simulink model "stopwatch_extended"  (R2020a)
settings: Solver=FixedStepAuto  StartTime=0.0  StopTime=1000.0  FixedStep=1e-3  RelTol=1e-3
settings Model: EnablePacing=on  Creator=Lukas Bilal  LastModifiedBy=Lukas Bilal

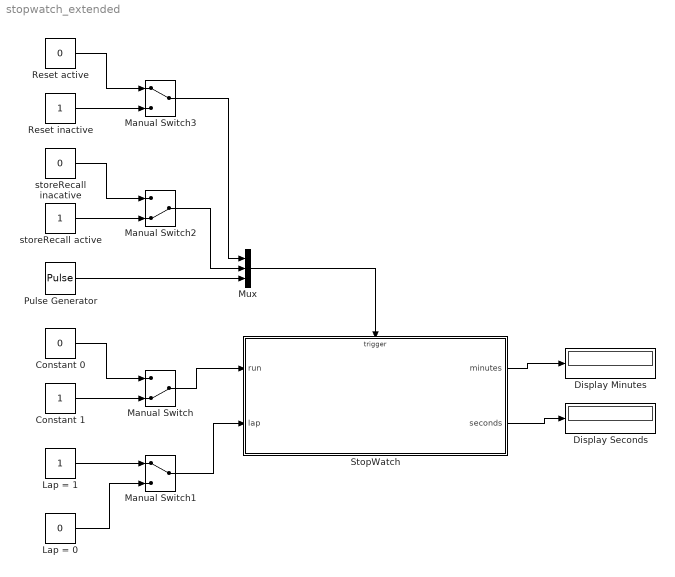
== system stopwatch_extended ==
  Constant 0 : Constant  Value=0  OutDataTypeStr=boolean
  Constant 1 : Constant  OutDataTypeStr=boolean
  Display Minutes : Display
  Display Seconds : Display
  Lap = 0 : Constant  Value=0  OutDataTypeStr=boolean
  Lap = 1 : Constant  OutDataTypeStr=boolean
  Manual Switch : ManualSwitch  CurrentSetting=0
  Manual Switch1 : ManualSwitch
  Manual Switch2 : ManualSwitch  CurrentSetting=0
  Manual Switch3 : ManualSwitch
  Mux : Mux  Inputs=3
  "Pulse Generator " : DiscretePulseGenerator  PulseType=Time based  Period=1  PulseWidth=5
  Reset active : Constant  Value=0  OutDataTypeStr=double
  Reset inactive : Constant  OutDataTypeStr=double
  StopWatch : Stateflow chart  TreatAsAtomicUnit=on
  storeRecall active : Constant  OutDataTypeStr=double
  storeRecall inacative : Constant  Value=0  OutDataTypeStr=double
  wires:
  "Pulse Generator "/1 -> Mux/3
  Constant 0/1 -> Manual Switch/1
  Constant 1/1 -> Manual Switch/2
  Manual Switch/1 -> StopWatch/1(run)
  StopWatch/1(minutes) -> Display Minutes/1
  StopWatch/2(seconds) -> Display Seconds/1
  Lap = 1/1 -> Manual Switch1/1
  Lap = 0/1 -> Manual Switch1/2
  Manual Switch1/1 -> StopWatch/2(lap)
  Mux/1 -> StopWatch/Trigger
  storeRecall inacative/1 -> Manual Switch2/1
  storeRecall active/1 -> Manual Switch2/2
  Manual Switch2/1 -> Mux/2
  Reset active/1 -> Manual Switch3/1
  Reset inactive/1 -> Manual Switch3/2
  Manual Switch3/1 -> Mux/1

== stateflow chart stopwatch_extended/StopWatch ==
  settings: executeAtInitialization=1
  state Stopped
    state Recall
    state Reset
    state Store
    (default) -> Recall
    Recall -> Reset [order 2] : Restart
    Store -> Recall [order 1] : storeRecall /
        | {
        |   minutes_intern = 0;
        |   seconds_intern = 0;
        |   seconds_stored = 0;
        |   minutes_stored = 0;
        | }
    Recall -> Store [order 1] : storeRecall /
        | {
        |   minutes_stored = minutes_intern;
        |   seconds_stored = seconds_intern;
        | }
    Reset -> Reset : {
        |   minutes_intern = 0;
        |   seconds_intern = 0;
        |   seconds_stored = 0;
        |   minutes_stored = 0;
        | }
    Store -> Reset [order 2] : Restart
  state Started
    state store_recall [parallel]
      settings: executionOrder=1
      (history)
      state recall
      state store
      (default) -> recall
      store -> recall : storeRecall /
          | {
          |   seconds_intern = seconds_stored;
          |   minutes_intern = minutes_stored;
          | }
      recall -> store : storeRecall /
          | {
          |   seconds_stored = seconds_intern;
          |   minutes_stored = minutes_intern;
          | }
    state Lap [parallel]
      settings: executionOrder=3
      state lap
      (default) -> lap
      lap -> lap : [lap] /
          | {
          |   seconds = seconds_intern;
          |   minutes = minutes_intern;
          | }
    state Counter [parallel]
      settings: executionOrder=2
      state Counter /
        on clk (seconds_intern == 59):
        minutes_intern = minutes_intern + 1;
        seconds_intern = seconds_intern + 1;
        on clk (seconds_intern < 59):
        seconds_intern = seconds_intern + 1;
      (default) -> Counter 
  (default) -> Stopped
  Stopped -> Started : [run] /
      | {
      |   seconds_intern = 0;
      |   minutes_intern = 0;
      | }
  Started -> Stopped : [~run]
  data: minutes output uint32; seconds output uint8; run input boolean; lap input boolean; minutes_intern local uint32; seconds_intern local uint8; seconds_stored local uint8; minutes_stored local uint32
  events: clk input RISING_EDGE_EVENT; storeRecall input RISING_EDGE_EVENT; Restart input RISING_EDGE_EVENT
